simulink library "RASPlib"  (R2015a)
settings: Solver=ode45  StartTime=0.0  StopTime=10.0  RelTol=1e-3
PostLoadFcn:
  | setsysloc(bdroot)
StartFcn:
  | open_system('MinSegLibrary','force')
libraries: arduinolib x7, simulink x3
settings Model: Creator=hurstj  LastModifiedBy=hurstj
settings DataIOCC: SignalLoggingSaveFormat=ModelDataLogs
settings DebuggingCC: UnderspecifiedInitializationDetection=Classic  MergeDetectMultiDrivingBlocksExec=none  SolverPrmCheckMsg=warning  MultiTaskDSMMsg=warning  MultiTaskCondExecSysMsg=none  StateNameClashWarn=warning  StrictBusMsg=None

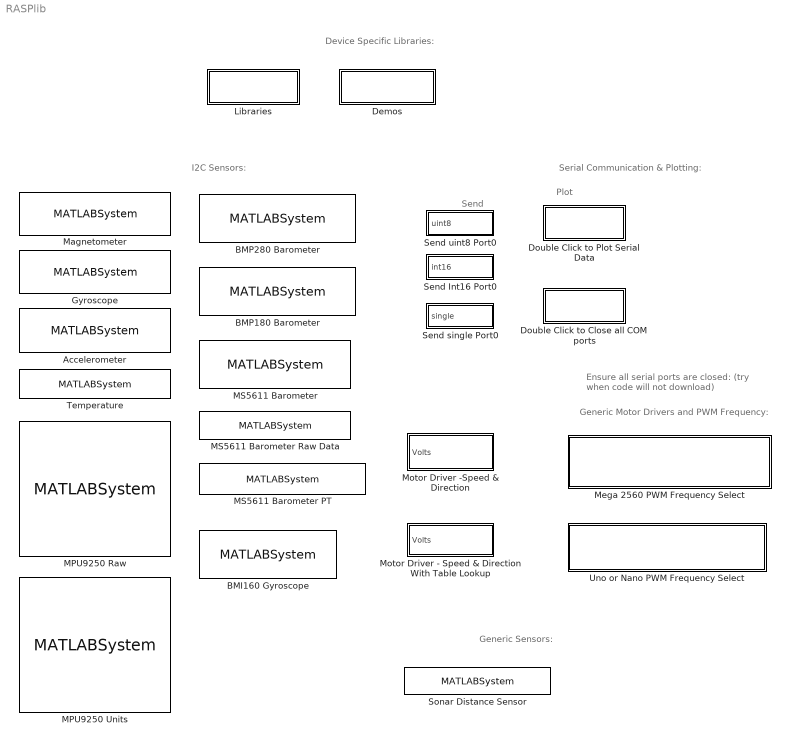
== system RASPlib ==
  note: Ensure all serial ports are closed:
      | (try when code will not download)
  note: Plot
  note: Send
  note: Device Specific Libraries:
  note: I2C Sensors:
  note: Serial Communication & Plotting:
  note: Generic Motor Drivers and PWM Frequency:
  note: Generic Sensors:
  Accelerometer : MATLABSystem  System=soMPU6050Accel  SimulateUsing=Code generation
      mask Type: soMPU6050Accel
      mask Display:
      | disp('soMPU6050Accel');
      | port_label('output',1,'xaccel');
      | port_label('output',2,'yaccel');
      | port_label('output',3,'zaccel');
  BMI160 Gyroscope : MATLABSystem  System=soBMI160Gyro
      mask Type: soBMI160Gyro
      mask Display:
      | disp('soBMI160Gyro');
      | port_label('output',1,'xvel');
      | port_label('output',2,'yvel');
      | port_label('output',3,'zvel');
  BMP180 Barometer : MATLABSystem  System=soBMP180  SimulateUsing=Code generation
      mask Type: soBMP180
      mask Display:
      | disp('soBMP180');
      | port_label('output',1,'pres_Pa');
      | port_label('output',2,'absAlt_m');
      | port_label('output',3,'temp_C');
  BMP280 Barometer : MATLABSystem  System=soBMP280  SimulateUsing=Code generation
      mask Type: soBMP280
      mask Display:
      | disp('soBMP280');
      | port_label('output',1,'pres_Pa');
      | port_label('output',2,'absAlt_m');
      | port_label('output',3,'temp_C');
  Demos : Subsystem
      settings: OpenFcn=Examples
      mask DialogControl DescTextVar Prompt: hello description
      mask Display: disp('OpenDemo')
  Double Click to Close all COM ports : Subsystem
      settings: OpenFcn=|
      | g=msgbox('Closing all COM ports');
      | disp('closing all COM ports')
      | newobjs=instrfindall
      | % Close them!
      | try,
      |     fclose(newobjs);
      |     delete(newobjs);
      | catch, end
      | pause(1), close(g);
      mask DialogControl DescTextVar Prompt: hello description
      mask Display: disp('CloseCOM')
  Double Click to Plot Serial Data : Subsystem  mask{COMport=28, BaudRate=9600, NumSamples=500, DataType=single, Ncx=1}
      mask prompts: COMport "COM Port:"; BaudRate "Baud Rate (needs to be same as Baud Rate in configuration parameters)"; NumSamples "Number of samples to plot"; DataType "Data Type of data being sent"; Ncx "N - Number of muxed channels"
      mask TypeOptions DataType: uint8 | int16 | single
      mask DialogControl DescTextVar Prompt: Plot single or multiple channel data received from the serial line.  View Matlab command window for connection and plot information.  After stopping graph, the data is stored in the variables fdat and wdat in the workspace.  Both variables are also saved to the file fdat.mat in the current directory.  The ploting procedure can be modified by editing the file SerialPlot.m. For multiple channels see example in MinSegNano_Demo.slx. This block does download code to the hardware - it sends the string '***Data Start***' before data is sent to help sync the data.  There should only be one of these blocks in the model.
      mask DialogControl Control2 Prompt: Click Here to Plot Data
      mask DialogControl Control2 Callback: SerialPlot(['COM' get_param(gcb,'COMport')], get_param(gcb,'DataType'), str2num(get_param(gcb,'NumSamples')), str2num(get_param(gcb,'BaudRate')),str2num(get_param(gcb,'Ncx')))
      mask Display: disp('SerialPlot')
  Gyroscope : MATLABSystem  System=soMPU6050Gyro  DLPFmode=0
      mask Type: soMPU6050Gyro
      mask Display:
      | disp('soMPU6050Gyro');
      | port_label('output',1,'xvel');
      | port_label('output',2,'yvel');
      | port_label('output',3,'zvel');
  Libraries : Subsystem
      settings: OpenFcn=HardwareLibraries
      mask DialogControl DescTextVar Prompt: hello description
      mask Display: disp('OpenLibrary')
  MPU9250 Raw : MATLABSystem  System=soMPU9250RAW  SimulateUsing=Code generation
      mask Type: soMPU9250RAW
      mask Display:
      | disp('soMPU9250RAW');
      | port_label('output',1,'xaccel');
      | port_label('output',2,'yaccel');
      | port_label('output',3,'zaccel');
      | port_label('output',4,'xgyro');
      | port_label('output',5,'ygyro');
      | port_label('output',6,'zgyro');
      | port_label('output',7,'xmag');
      | port_label('output',8,'ymag');
      | port_label('output',9,'zmag');
      | port_label('output',10,'temp');
  MPU9250 Units : MATLABSystem  System=soMPU9250  SimulateUsing=Code generation
      mask Type: soMPU9250
      mask Display:
      | disp('soMPU9250');
      | port_label('output',1,'ax_mg');
      | port_label('output',2,'ay_mg');
      | port_label('output',3,'az_mg');
      | port_label('output',4,'gx_ds');
      | port_label('output',5,'gy_ds');
      | port_label('output',6,'gz_ds');
      | port_label('output',7,'mx_mG');
      | port_label('output',8,'my_mG');
      | port_label('output',9,'mz_mG');
      | port_label('output',10,'temp_C');
  MS5611 Barometer : MATLABSystem  System=soMS5611  SimulateUsing=Code generation
      mask Type: soMS5611
      mask Display:
      | disp('soMS5611');
      | port_label('output',1,'pres_Pa');
      | port_label('output',2,'temp_C');
      | port_label('output',3,'absAlt_m');
      | port_label('output',4,'relAlt_m');
  MS5611 Barometer PT : MATLABSystem  System=soMS5611BaroPT  SimulateUsing=Code generation
      mask Type: soMS5611BaroPT
      mask Display:
      | disp('soMS5611BaroPT');
      | port_label('output',1,'pres_Pa');
      | port_label('output',2,'temp_C');
  MS5611 Barometer Raw Data : MATLABSystem  System=soMS5611BaroRAW  SimulateUsing=Code generation
      mask Type: soMS5611BaroRAW
      mask Display:
      | disp('soMS5611BaroRAW');
      | port_label('output',1,'pres');
      | port_label('output',2,'temp');
  Magnetometer : MATLABSystem  System=soHMC5883L  SimulateUsing=Code generation
      mask Type: soHMC5883L
      mask Display:
      | disp('soHMC5883L');
      | port_label('output',1,'xmag');
      | port_label('output',2,'ymag');
      | port_label('output',3,'zmag');
  Mega 2560 PWM Frequency Select : Subsystem  mask{Frequency=32KHz, Timer=4 - pins 6, 7, 8}
      mask help:
      | Selects the Mega 2560 PWM frequency based on the timer for the pin:
      |
      | Timer 1: pins 11, 12
      | Timer 2: pins 9, 10
      | Timer 3: pins 2, 3, 5
      | Timer 4: pins 6, 7, 8
      | Timer 5: pins 44, 45, 46
      |
      | Does not do Timer 0: pins 4, 13, since timer 0 affects major timing events.
      |
      | Frequiencies 32000Hz, 4000KHz, 490Hz, 122Hz, 30Hz corresponding to divisor 1, 8, 64, 256, 1024
      mask TypeOptions Frequency: 32KHz | 4KHz | 490Hz | 122Hz | 30Hz
      mask TypeOptions Timer: 1 - pins 11, 12 | 2 - pins 9, 10 | 3 - pins 2, 3, 5 | 4 - pins 6, 7, 8 | 5 - pins 44, 45, 46
      mask Display:
      | switch Frequency
      |     case 1, f='32KHz';
      |     case 2, f='4KHz';
      |     case 3, f='490Hz';
      |     case 4, f='122Hz';
      |     case 5, f='30Hz';
      | end
      | switch Timer
      |     case 1, t='pins 11, 12';
      |     case 2, t='pins 9, 10';
      |     case 3, t='pins 2, 3, 5';
      |     case 4, t='pins 6, 7, 8';
      |     case 5, t='pins 44, 45, 45';
      | end
      | fprintf('Mega 2560 PWM Frequency Select')
      | fprintf(['\n\n' t , ' Frequency '  f], t)
  Motor Driver - Speed & Direction With Table Lookup : Subsystem  mask(Motor Driver){Vsupply=3.25, Direction=1, PWMPin=5, DigitalPin=4}
      mask prompts: Vsupply "Driver Voltage"; PWMPin "PWM Pin"; DigitalPin "Digital Pin"
      mask help:
      | Use a single PWM and a single Digtial out to control the magnitude and direction of a motor.  A lookup table is implemented to allow correction of a nonliear PWM to voltage map.
      |
      | Specify driver supply voltage (3.25 for USB with SN754410)
      | Direction can be -1 to reverse the motor direction
      mask Display:
      | port_label('input',1,'Volts')
      | text(15,5,['Vsupply=' num2str(Vsupply)])
  Motor Driver -Speed & Direction : Subsystem  mask(Motor Driver){Vsupply=3.25, PWMPin=5, DigitalPin=4}
      mask prompts: Vsupply "Driver Voltage"; PWMPin "PWM Pin"; DigitalPin "Digital Pin"
      mask help:
      | Use a single PWM and a single Digtial out to control the magnitude and direction of a motor
      |
      | Specify driver supply voltage (3.25 for USB with SN754410)
      mask Display:
      | port_label('input',1,'Volts')
      | text(15,5,['Vsupply=' num2str(Vsupply)])
  Send Int16 Port0 : Subsystem
  Send single Port0 : Subsystem
  Send uint8 Port0 : Subsystem
  Sonar Distance Sensor : MATLABSystem  System=soHCSR04Sonar  Sonar=1  TrigPin=7  EchoPin=8
      mask Type: soHCSR04Sonar
      mask Display:
      | disp('soHCSR04Sonar');
      | port_label('output',1,'d_cm');
  Temperature : MATLABSystem  System=soMPU6050Temp  SimulateUsing=Code generation
      mask Type: soMPU6050Temp
      mask Display:
      | disp('soMPU6050Temp');
      | port_label('output',1,'temp');
  Uno or Nano PWM Frequency Select : Subsystem  mask{Frequency=4KHz, Timer=1 - pins 9, 10}
      mask help:
      | Selects the ATmega328P PWM frequency based on the timer for the pin:
      |
      | Timer 1: pins 9, 10
      | Timer 2: pins 3, 11
      |
      | Does not do Timer 0: pins 5, 6, since timer 0 affects major timing events.
      |
      | Frequiencies 32000Hz, 4000KHz, 490Hz, 122Hz, 30Hz corresponding to divisor 1, 8, 64, 256, 1024
      mask TypeOptions Frequency: 32KHz | 4KHz | 490Hz | 122Hz | 30Hz
      mask TypeOptions Timer: 1 - pins 9, 10 | 2 - pins 3, 11
      mask Display:
      | switch Frequency
      |     case 1, f='32KHz';
      |     case 2, f='4KHz';
      |     case 3, f='490Hz';
      |     case 4, f='122Hz';
      |     case 5, f='30Hz';
      | end
      | switch Timer
      |     case 1, t='pins 9, 10';
      |     case 2, t='pins 3, 11';
      | end
      | fprintf('ATmega328P PWM Frequency Select')
      | fprintf(['\n\n' t , ' Frequency '  f], t)

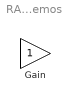
== system RASPlib/Demos ==
  Gain : Gain

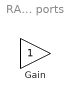
== system RASPlib/Double Click to Close all COM ports ==
  Gain : Gain

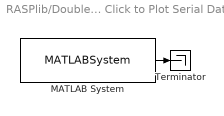
== system RASPlib/Double Click to Plot Serial Data ==
  MATLAB System : MATLABSystem  System=soSendDataStartString  SampleTime=0.1
      mask Type: soSendDataStartString
      mask Display:
      | disp('Send Data Start String');
      | port_label('output',1,'y');
  Terminator : Terminator
  wires:
  MATLAB System/1 -> Terminator/1

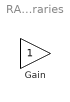
== system RASPlib/Libraries ==
  Gain : Gain

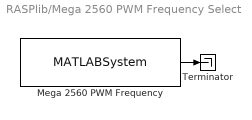
== system RASPlib/Mega 2560 PWM Frequency Select ==
  Mega 2560 PWM Frequency : MATLABSystem  System=PWMselect  PWMFSelect=Frequency  PWMTimer=Timer  SampleTime=0
      mask Type: PWMselect
      mask Display:
      | disp('Mega PWM Frequency Select');
      | port_label('output',1,'y');
  Terminator : Terminator
  wires:
  Mega 2560 PWM Frequency/1 -> Terminator/1

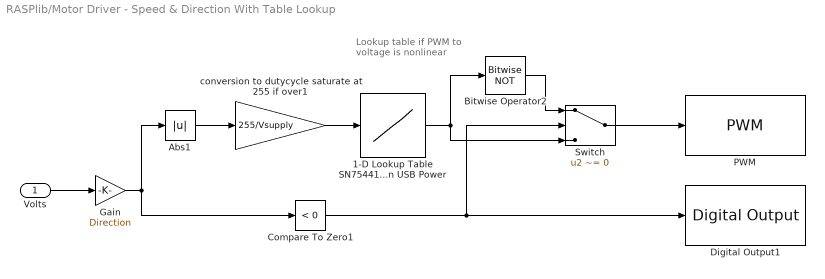
== system RASPlib/Motor Driver - Speed & Direction With Table Lookup ==
  note: Lookup table if
      | PWM to voltage
      | is nonlinear
  Volts : Inport
  1-D Lookup Table SN754410 Maxon USB Power : Lookup_n-D  NumberOfTableDimensions=1  BreakpointsForDimension1=[0 3 110 255]  BreakpointsForDimension1DataTypeStr=uint8  Table=[0 13 28 255]  TableDataTypeStr=uint8  ExtrapMethod=Clip  UseLastTableValue=on  InternalRulePriority=Speed  OutDataTypeStr=uint8  RndMeth=Simplest  SaturateOnIntegerOverflow=on  InputSameDT=on
  Abs1 : Abs
  Bitwise Operator2 : simulink/Logic and Bit Operations/Bitwise Operator  logicop=NOT  UseBitMask=off  BitMask=bin2dec('11011001')  BitMaskRealWorld=Stored Integer
  Compare To Zero1 : simulink/Logic and Bit Operations/Compare To Zero  relop=<  OutDataTypeStr=boolean
  Digital Output1 : arduinolib/Digital Output  pinNumber=DigitalPin  blockPlatform=arduino
  Gain : Gain  Gain=Direction
  PWM : arduinolib/PWM  pinNumber=PWMPin  blockPlatform=arduino
  Switch : Switch  Criteria=u2 ~= 0
  conversion to dutycycle saturate at 255 if over1 : Gain  Gain=255/Vsupply  OutDataTypeStr=uint8  SaturateOnIntegerOverflow=on
  wires:
  Compare To Zero1/1 -> Digital Output1/1, Switch/2
  conversion to dutycycle saturate at 255 if over1/1 -> 1-D Lookup Table SN754410 Maxon USB Power/1
  Volts/1 -> Gain/1
  Abs1/1 -> conversion to dutycycle saturate at 255 if over1/1
  Switch/1 -> PWM/1
  1-D Lookup Table SN754410 Maxon USB Power/1 -> Switch/3, Bitwise Operator2/1
  Bitwise Operator2/1 -> Switch/1
  Gain/1 -> Compare To Zero1/1, Abs1/1

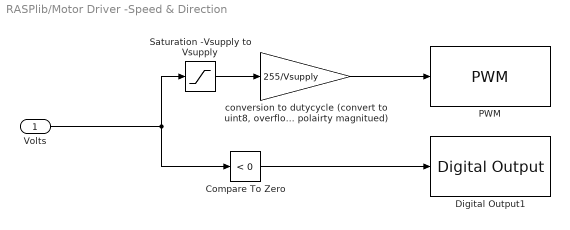
== system RASPlib/Motor Driver -Speed & Direction ==
  Volts : Inport
  Compare To Zero : simulink/Logic and Bit Operations/Compare To Zero  relop=<  OutDataTypeStr=boolean
  Digital Output1 : arduinolib/Digital Output  pinNumber=DigatlPin  blockPlatform=arduino
  PWM : arduinolib/PWM  pinNumber=PWMPin  blockPlatform=arduino
  Saturation -Vsupply to Vsupply : Saturate  UpperLimit=Vsupply  LowerLimit=-Vsupply  OutDataTypeStr=single
  "conversion to dutycycle (convert to uint8, overflow will provide reverse polairty magnitued)" : Gain  Gain=255/Vsupply  OutDataTypeStr=uint8
  wires:
  Compare To Zero/1 -> Digital Output1/1
  "conversion to dutycycle (convert to uint8, overflow will provide reverse polairty magnitued)"/1 -> PWM/1
  Saturation -Vsupply to Vsupply/1 -> "conversion to dutycycle (convert to uint8, overflow will provide reverse polairty magnitued)"/1
  Volts/1 -> Saturation -Vsupply to Vsupply/1, Compare To Zero/1

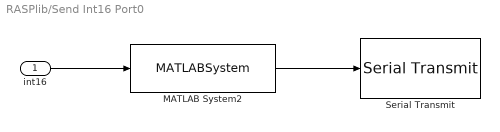
== system RASPlib/Send Int16 Port0 ==
  int16 : Inport
  MATLAB System2 : MATLABSystem  System=so_int2bytes  SimulateUsing=Code generation
      mask Type: so_int2bytes
      mask Display:
      | disp('so_int2bytes');
      | port_label('input',1,'int_in');
      | port_label('output',1,'out');
  Serial Transmit : arduinolib/Serial Transmit  portNumber=0  blockPlatform=arduino
  wires:
  MATLAB System2/1 -> Serial Transmit/1
  int16/1 -> MATLAB System2/1

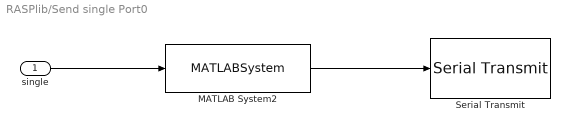
== system RASPlib/Send single Port0 ==
  single : Inport  OutDataTypeStr=single  LockScale=on
  MATLAB System2 : MATLABSystem  System=so_float2bytes  SimulateUsing=Code generation
      mask Type: so_float2bytes
      mask Display:
      | disp('so_float2bytes');
      | port_label('input',1,'fin');
      | port_label('output',1,'out');
  Serial Transmit : arduinolib/Serial Transmit  portNumber=0  blockPlatform=arduino
  wires:
  single/1 -> MATLAB System2/1
  MATLAB System2/1 -> Serial Transmit/1

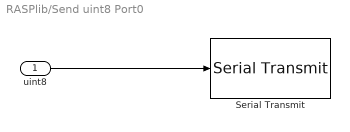
== system RASPlib/Send uint8 Port0 ==
  uint8 : Inport
  Serial Transmit : arduinolib/Serial Transmit  portNumber=0  blockPlatform=arduino
  wires:
  uint8/1 -> Serial Transmit/1

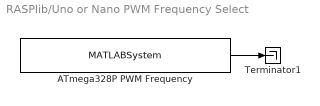
== system RASPlib/Uno or Nano PWM Frequency Select ==
  ATmega328P PWM Frequency : MATLABSystem  System=PWMselect_uno_nano  PWMFSelect=Frequency  PWMTimer=Timer  SampleTime=0
      mask Type: PWMselect_uno_nano
      mask Display:
      | disp('ATmega328P PWM Frequency Select');
      | port_label('output',1,'y');
  Terminator1 : Terminator
  wires:
  ATmega328P PWM Frequency/1 -> Terminator1/1
